simulink model "morphological_operations"  (Simulink 7.9)
settings: Solver=FixedStepDiscrete  StartTime=0.0  StopTime=0.0  RelTol=1e-3
undefined symbols (not defined in the file or in its folder): jet, strel
libraries: visionsinks x5, visionmorphops x4, visionsources x1
settings Model: Creator=lenovo  LastModifiedBy=lenovo
settings DebuggingCC: SolverPrmCheckMsg=none

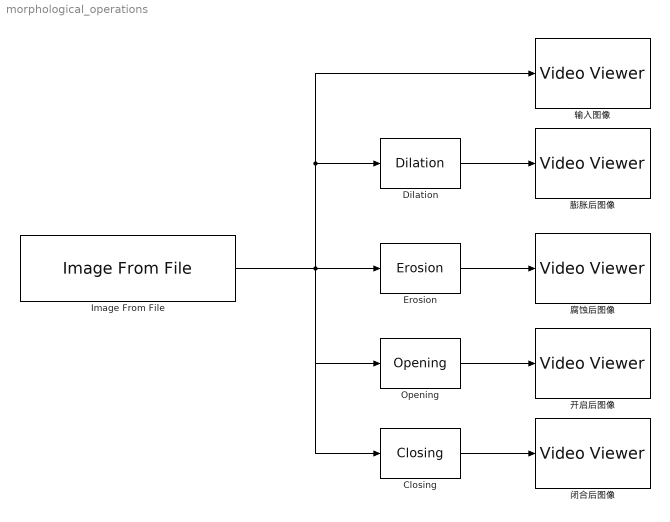
== system morphological_operations ==
  Closing : visionmorphops/Closing  nhoodsrc=Specify via dialog  strel=strel('line',5,45)
  Dilation : visionmorphops/Dilation  nhoodsrc=Specify via dialog  strel=[1 1; 1 1]
  Erosion : visionmorphops/Erosion  nhoodsrc=Specify via dialog  strel=strel('square',4)
  Image From File : visionsources/Image From File  Tag=vipblks_nd  FileName=cameraman.tif  imagePorts=One multidimensional signal  Ts=inf  ImageDataType=Inherit from input image  Signed=on  WordLength=16  sdImageDataType=uint(8)  FractionLengthMode=User-defined  FractionLength=15  OutPortLabels=R|G|B
  Opening : visionmorphops/Opening  nhoodsrc=Specify via dialog  strel=strel('disk',5)
  开启后图像 : visionsinks/Video Viewer  inputType=Obsolete7b  imagePorts=One multidimensional signal  useColorMap=off  colormapValue=jet(256)  specRange=off  minInputVal=0  maxInputVal=255  FigPos=[478 533 410 300]  AxisZoom=on  trueSizedOnce=off  OpenAtMdlStart=on
  腐蚀后图像 : visionsinks/Video Viewer  inputType=Obsolete7b  imagePorts=One multidimensional signal  useColorMap=off  colormapValue=jet(256)  specRange=off  minInputVal=0  maxInputVal=255  FigPos=[575 696 512 394]  AxisZoom=on  trueSizedOnce=off  OpenAtMdlStart=on
  膨胀后图像 : visionsinks/Video Viewer  inputType=Obsolete7b  imagePorts=One multidimensional signal  useColorMap=off  colormapValue=jet(256)  specRange=off  minInputVal=0  maxInputVal=255  FigPos=[654 590 410 300]  AxisZoom=on  trueSizedOnce=off  OpenAtMdlStart=on
  输入图像 : visionsinks/Video Viewer  inputType=Obsolete7b  imagePorts=One multidimensional signal  useColorMap=off  colormapValue=jet(256)  specRange=off  minInputVal=0  maxInputVal=255  FigPos=[-1 678 410 300]  AxisZoom=on  trueSizedOnce=off  OpenAtMdlStart=on
  闭合后图像 : visionsinks/Video Viewer  inputType=Obsolete7b  imagePorts=One multidimensional signal  useColorMap=off  colormapValue=jet(256)  specRange=off  minInputVal=0  maxInputVal=255  FigPos=[-64 533 410 300]  AxisZoom=on  trueSizedOnce=off  OpenAtMdlStart=on
  wires:
  Image From File/1 -> 输入图像/1, Dilation/1, Opening/1, Erosion/1, Closing/1
  Erosion/1 -> 腐蚀后图像/1
  Opening/1 -> 开启后图像/1
  Closing/1 -> 闭合后图像/1
  Dilation/1 -> 膨胀后图像/1
